simulink model "TST_Fans_ClgDem"  (R2016b)
settings: Solver=FixedStepDiscrete  StartTime=0.0  StopTime=simTime  FixedStep=sampleTime  RelTol=1e-3
values from neighbouring files (symbols this model uses):
  testCase = 1    [initTST_Fans_ClgDem_001.m]
libraries: simulink x4, UnitTest_Lib x2
settings Model: Creator=xinchangran  LastModifiedBy=xinchangran
settings DebuggingCC: SignalRangeChecking=error

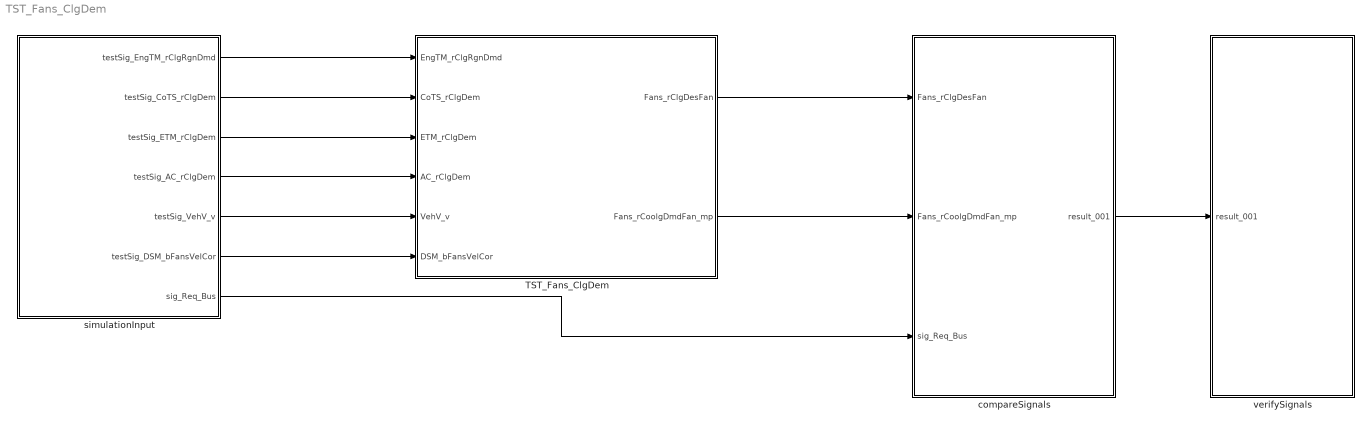
== system TST_Fans_ClgDem ==
  TST_Fans_ClgDem : Subsystem
  compareSignals : Subsystem
  simulationInput : Subsystem
  verifySignals : Subsystem
  wires:
  simulationInput/1(testSig_EngTM_rClgRgnDmd) -> TST_Fans_ClgDem/1(EngTM_rClgRgnDmd)
  simulationInput/2(testSig_CoTS_rClgDem) -> TST_Fans_ClgDem/2(CoTS_rClgDem)
  simulationInput/3(testSig_ETM_rClgDem) -> TST_Fans_ClgDem/3(ETM_rClgDem)
  simulationInput/4(testSig_AC_rClgDem) -> TST_Fans_ClgDem/4(AC_rClgDem)
  simulationInput/5(testSig_VehV_v) -> TST_Fans_ClgDem/5(VehV_v)
  simulationInput/6(testSig_DSM_bFansVelCor) -> TST_Fans_ClgDem/6(DSM_bFansVelCor)
  TST_Fans_ClgDem/1(Fans_rClgDesFan) -> compareSignals/1(Fans_rClgDesFan)
  TST_Fans_ClgDem/2(Fans_rCoolgDmdFan_mp) -> compareSignals/2(Fans_rCoolgDmdFan_mp)
  simulationInput/7(sig_Req_Bus) -> compareSignals/3(sig_Req_Bus)
  compareSignals/1(result_001) -> verifySignals/1(result_001)

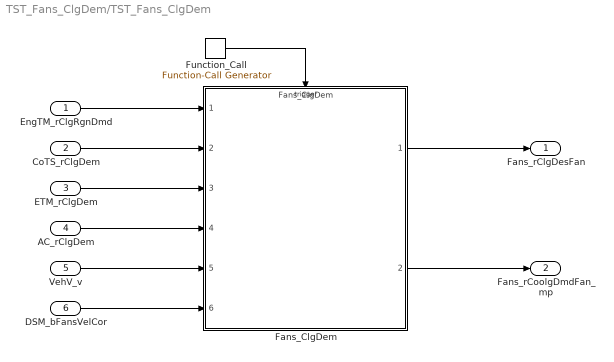
== system TST_Fans_ClgDem/TST_Fans_ClgDem ==
  EngTM_rClgRgnDmd : Inport
  CoTS_rClgDem : Inport  Port=2
  ETM_rClgDem : Inport  Port=3
  AC_rClgDem : Inport  Port=4
  VehV_v : Inport  Port=5
  DSM_bFansVelCor : Inport  Port=6
  Fans_ClgDem : ModelReference  ModelNameDialog=Fans_ClgDem  SimulationMode=Normal  ModelReferenceVersion=1.39  TriggerPortName=function  TriggerPortTriggerType=function-call  TriggerPortStatesWhenEnabling=held
  Function_Call : simulink/Ports & Subsystems/Function-Call Generator  sample_time=sampleTime  numberOfIterations=1
  Fans_rClgDesFan : Outport
  Fans_rCoolgDmdFan_mp : Outport  Port=2
  wires:
  Function_Call/1 -> Fans_ClgDem/Trigger
  EngTM_rClgRgnDmd/1 -> Fans_ClgDem/1
  CoTS_rClgDem/1 -> Fans_ClgDem/2
  ETM_rClgDem/1 -> Fans_ClgDem/3
  AC_rClgDem/1 -> Fans_ClgDem/4
  VehV_v/1 -> Fans_ClgDem/5
  DSM_bFansVelCor/1 -> Fans_ClgDem/6
  Fans_ClgDem/1 -> Fans_rClgDesFan/1
  Fans_ClgDem/2 -> Fans_rCoolgDmdFan_mp/1

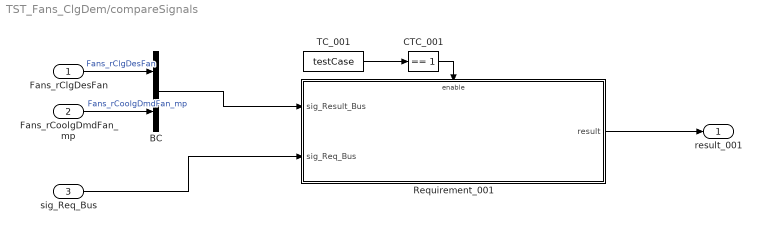
== system TST_Fans_ClgDem/compareSignals ==
  Fans_rClgDesFan : Inport
  Fans_rCoolgDmdFan_mp : Inport  Port=2
  sig_Req_Bus : Inport  Port=3
  BC : BusCreator  Inputs=2
  CTC_001 : simulink/Logic and Bit Operations/Compare To Constant  relop===  const=1  OutDataTypeStr=boolean
  Requirement_001 : Subsystem
  TC_001 : Constant  Value=testCase
  result_001 : Outport
  wires:
  Fans_rClgDesFan/1 -> BC/1  "Fans_rClgDesFan"
  Fans_rCoolgDmdFan_mp/1 -> BC/2  "Fans_rCoolgDmdFan_mp"
  TC_001/1 -> CTC_001/1
  CTC_001/1 -> Requirement_001/Enable
  sig_Req_Bus/1 -> Requirement_001/2(sig_Req_Bus)
  BC/1 -> Requirement_001/1(sig_Result_Bus)
  Requirement_001/1(result) -> result_001/1

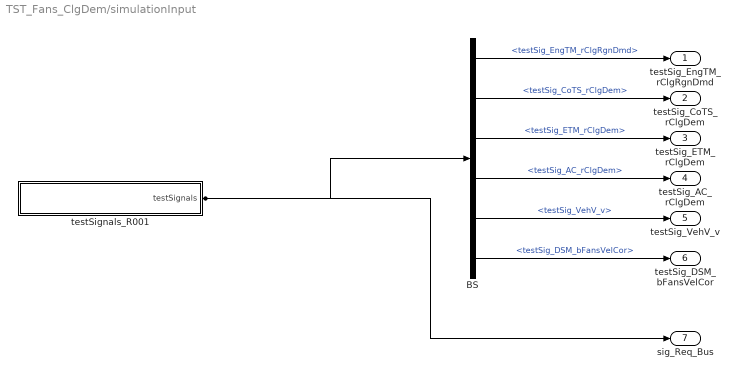
== system TST_Fans_ClgDem/simulationInput ==
  BS : BusSelector  OutputSignals=testSig_EngTM_rClgRgnDmd,testSig_CoTS_rClgDem,testSig_ETM_rClgDem,testSig_AC_rClgDem,testSig_VehV_v,testSig_DSM_bFansVelCor
  testSignals_R001 : Subsystem
  testSig_EngTM_rClgRgnDmd : Outport
  testSig_CoTS_rClgDem : Outport  Port=2
  testSig_ETM_rClgDem : Outport  Port=3
  testSig_AC_rClgDem : Outport  Port=4
  testSig_VehV_v : Outport  Port=5
  testSig_DSM_bFansVelCor : Outport  Port=6
  sig_Req_Bus : Outport  Port=7
  wires:
  BS/1 -> testSig_EngTM_rClgRgnDmd/1  "<testSig_EngTM_rClgRgnDmd>"
  BS/2 -> testSig_CoTS_rClgDem/1  "<testSig_CoTS_rClgDem>"
  BS/3 -> testSig_ETM_rClgDem/1  "<testSig_ETM_rClgDem>"
  BS/4 -> testSig_AC_rClgDem/1  "<testSig_AC_rClgDem>"
  BS/5 -> testSig_VehV_v/1  "<testSig_VehV_v>"
  BS/6 -> testSig_DSM_bFansVelCor/1  "<testSig_DSM_bFansVelCor>"
  testSignals_R001/1(testSignals) -> BS/1, sig_Req_Bus/1

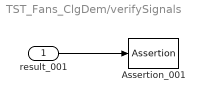
== system TST_Fans_ClgDem/verifySignals ==
  result_001 : Inport
  Assertion_001 : Assertion  Enabled=off
  wires:
  result_001/1 -> Assertion_001/1

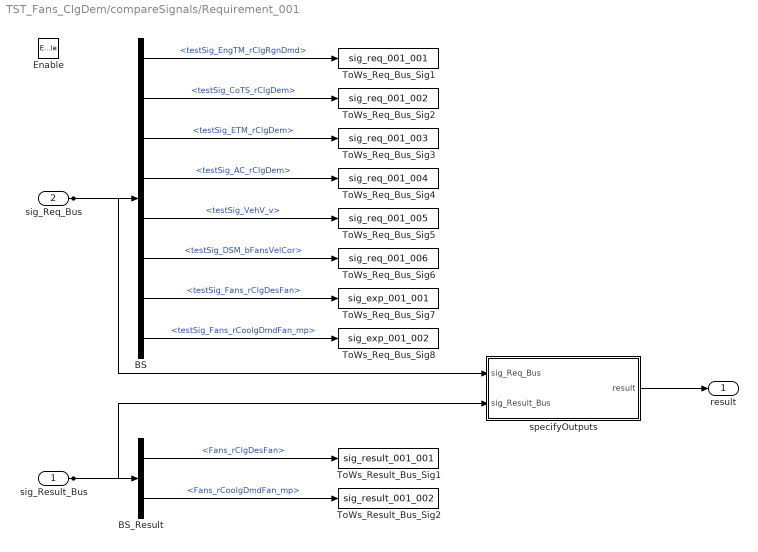
== system TST_Fans_ClgDem/compareSignals/Requirement_001 ==
  sig_Result_Bus : Inport
  sig_Req_Bus : Inport  Port=2
  Enable : EnablePort
  BS : BusSelector  OutputSignals=testSig_EngTM_rClgRgnDmd,testSig_CoTS_rClgDem,testSig_ETM_rClgDem,testSig_AC_rClgDem,testSig_VehV_v,testSig_DSM_bFansVelCor,testSig_Fans_rClgDesFan,testSig_Fans_rCoolgDmdFan_mp
  BS_Result : BusSelector  OutputSignals=Fans_rClgDesFan,Fans_rCoolgDmdFan_mp
  ToWs_Req_Bus_Sig1 : ToWorkspace  VariableName=sig_req_001_001  SaveFormat=Structure With Time
  ToWs_Req_Bus_Sig2 : ToWorkspace  VariableName=sig_req_001_002  SaveFormat=Structure With Time
  ToWs_Req_Bus_Sig3 : ToWorkspace  VariableName=sig_req_001_003  SaveFormat=Structure With Time
  ToWs_Req_Bus_Sig4 : ToWorkspace  VariableName=sig_req_001_004  SaveFormat=Structure With Time
  ToWs_Req_Bus_Sig5 : ToWorkspace  VariableName=sig_req_001_005  SaveFormat=Structure With Time
  ToWs_Req_Bus_Sig6 : ToWorkspace  VariableName=sig_req_001_006  SaveFormat=Structure With Time
  ToWs_Req_Bus_Sig7 : ToWorkspace  VariableName=sig_exp_001_001  SaveFormat=Structure With Time
  ToWs_Req_Bus_Sig8 : ToWorkspace  VariableName=sig_exp_001_002  SaveFormat=Structure With Time
  ToWs_Result_Bus_Sig1 : ToWorkspace  VariableName=sig_result_001_001  SaveFormat=Structure With Time
  ToWs_Result_Bus_Sig2 : ToWorkspace  VariableName=sig_result_001_002  SaveFormat=Structure With Time
  specifyOutputs : Subsystem
  result : Outport
  wires:
  sig_Req_Bus/1 -> BS/1, specifyOutputs/1(sig_Req_Bus)
  BS/1 -> ToWs_Req_Bus_Sig1/1  "<testSig_EngTM_rClgRgnDmd>"
  BS/2 -> ToWs_Req_Bus_Sig2/1  "<testSig_CoTS_rClgDem>"
  BS/3 -> ToWs_Req_Bus_Sig3/1  "<testSig_ETM_rClgDem>"
  BS/4 -> ToWs_Req_Bus_Sig4/1  "<testSig_AC_rClgDem>"
  BS/5 -> ToWs_Req_Bus_Sig5/1  "<testSig_VehV_v>"
  BS/6 -> ToWs_Req_Bus_Sig6/1  "<testSig_DSM_bFansVelCor>"
  BS/7 -> ToWs_Req_Bus_Sig7/1  "<testSig_Fans_rClgDesFan>"
  BS/8 -> ToWs_Req_Bus_Sig8/1  "<testSig_Fans_rCoolgDmdFan_mp>"
  sig_Result_Bus/1 -> BS_Result/1, specifyOutputs/2(sig_Result_Bus)
  BS_Result/1 -> ToWs_Result_Bus_Sig1/1  "<Fans_rClgDesFan>"
  BS_Result/2 -> ToWs_Result_Bus_Sig2/1  "<Fans_rCoolgDmdFan_mp>"
  specifyOutputs/1(result) -> result/1

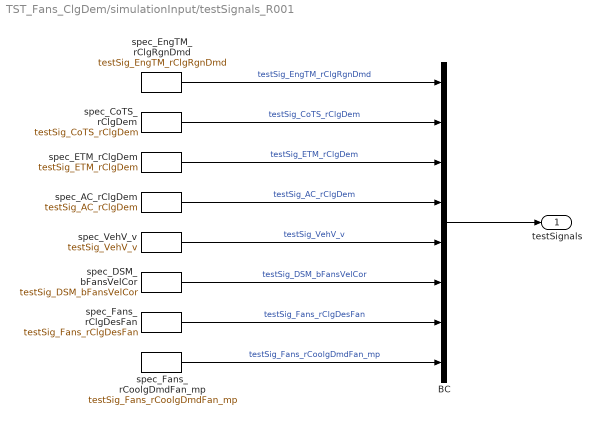
== system TST_Fans_ClgDem/simulationInput/testSignals_R001 ==
  BC : BusCreator  Inputs=8
  spec_AC_rClgDem : FromWorkspace  VariableName=testSig_AC_rClgDem  Interpolate=off  OutputAfterFinalValue=Holding final value
  spec_CoTS_rClgDem : FromWorkspace  VariableName=testSig_CoTS_rClgDem  Interpolate=off  OutputAfterFinalValue=Holding final value
  spec_DSM_bFansVelCor : FromWorkspace  VariableName=testSig_DSM_bFansVelCor  Interpolate=off  OutputAfterFinalValue=Holding final value
  spec_ETM_rClgDem : FromWorkspace  VariableName=testSig_ETM_rClgDem  Interpolate=off  OutputAfterFinalValue=Holding final value
  spec_EngTM_rClgRgnDmd : FromWorkspace  VariableName=testSig_EngTM_rClgRgnDmd  Interpolate=off  OutputAfterFinalValue=Holding final value
  spec_Fans_rClgDesFan : FromWorkspace  VariableName=testSig_Fans_rClgDesFan  Interpolate=off  OutputAfterFinalValue=Holding final value
  spec_Fans_rCoolgDmdFan_mp : FromWorkspace  VariableName=testSig_Fans_rCoolgDmdFan_mp  Interpolate=off  OutputAfterFinalValue=Holding final value
  spec_VehV_v : FromWorkspace  VariableName=testSig_VehV_v  Interpolate=off  OutputAfterFinalValue=Holding final value
  testSignals : Outport
  wires:
  BC/1 -> testSignals/1
  spec_EngTM_rClgRgnDmd/1 -> BC/1  "testSig_EngTM_rClgRgnDmd"
  spec_CoTS_rClgDem/1 -> BC/2  "testSig_CoTS_rClgDem"
  spec_ETM_rClgDem/1 -> BC/3  "testSig_ETM_rClgDem"
  spec_AC_rClgDem/1 -> BC/4  "testSig_AC_rClgDem"
  spec_VehV_v/1 -> BC/5  "testSig_VehV_v"
  spec_DSM_bFansVelCor/1 -> BC/6  "testSig_DSM_bFansVelCor"
  spec_Fans_rClgDesFan/1 -> BC/7  "testSig_Fans_rClgDesFan"
  spec_Fans_rCoolgDmdFan_mp/1 -> BC/8  "testSig_Fans_rCoolgDmdFan_mp"

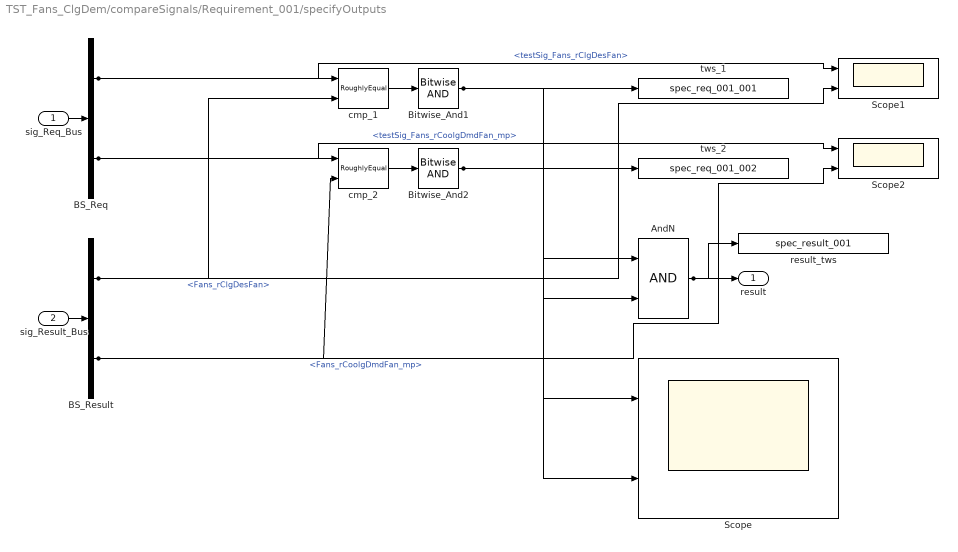
== system TST_Fans_ClgDem/compareSignals/Requirement_001/specifyOutputs ==
  sig_Req_Bus : Inport
  sig_Result_Bus : Inport  Port=2
  AndN : Logic
  BS_Req : BusSelector  OutputSignals=testSig_Fans_rClgDesFan,testSig_Fans_rCoolgDmdFan_mp
  BS_Result : BusSelector  OutputSignals=Fans_rClgDesFan,Fans_rCoolgDmdFan_mp
  Bitwise_And1 : simulink/Logic and Bit Operations/Bitwise Operator  logicop=AND  UseBitMask=off  BitMask=bin2dec('11011001')  BitMaskRealWorld=Stored Integer
  Bitwise_And2 : simulink/Logic and Bit Operations/Bitwise Operator  logicop=AND  UseBitMask=off  BitMask=bin2dec('11011001')  BitMaskRealWorld=Stored Integer
  Scope : Scope  NumInputPorts=2
  Scope1 : Scope  NumInputPorts=2
  Scope2 : Scope  NumInputPorts=2
  cmp_1 : UnitTest_Lib/RoughlyEqual  slope=0.1
  cmp_2 : UnitTest_Lib/RoughlyEqual  slope=0.1
  result_tws : ToWorkspace  VariableName=spec_result_001
  tws_1 : ToWorkspace  VariableName=spec_req_001_001
  tws_2 : ToWorkspace  VariableName=spec_req_001_002
  result : Outport
  wires:
  sig_Req_Bus/1 -> BS_Req/1
  sig_Result_Bus/1 -> BS_Result/1
  AndN/1 -> result/1, result_tws/1
  BS_Req/1 -> cmp_1/1, Scope1/1  "<testSig_Fans_rClgDesFan>"
  BS_Result/1 -> cmp_1/2, Scope1/2  "<Fans_rClgDesFan>"
  cmp_1/1 -> Bitwise_And1/1
  Bitwise_And1/1 -> tws_1/1, AndN/1, Scope/1
  BS_Req/2 -> cmp_2/1, Scope2/1  "<testSig_Fans_rCoolgDmdFan_mp>"
  BS_Result/2 -> cmp_2/2, Scope2/2  "<Fans_rCoolgDmdFan_mp>"
  cmp_2/1 -> Bitwise_And2/1
  Bitwise_And2/1 -> tws_2/1, AndN/2, Scope/2
